simulink model "sampleModel2019_4_sub_sub_sub"  (R2023a)
settings: Solver=VariableStepAuto  StartTime=0.0  StopTime=10.0  RelTol=1e-3
libraries: hdlsllib x6, simulink x2
settings Model: Creator=user1  LastModifiedBy=user1
settings OptimizationCC: BlockReduction=off  ConditionallyExecuteInputs=off

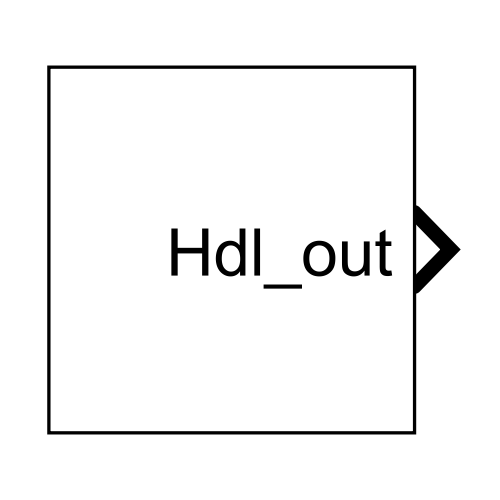
[thumbnail: Simulink's stored preview of the top-level diagram]
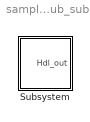
== system sampleModel2019_4_sub_sub_sub ==
  Subsystem : Subsystem

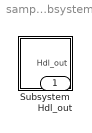
== system sampleModel2019_4_sub_sub_sub/Subsystem ==
  Subsystem : Subsystem
  Hdl_out : Outport  OutDataTypeStr=uint8

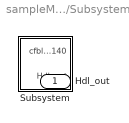
== system sampleModel2019_4_sub_sub_sub/Subsystem/Subsystem ==
  Subsystem : Subsystem
  Hdl_out : Outport  OutDataTypeStr=uint8

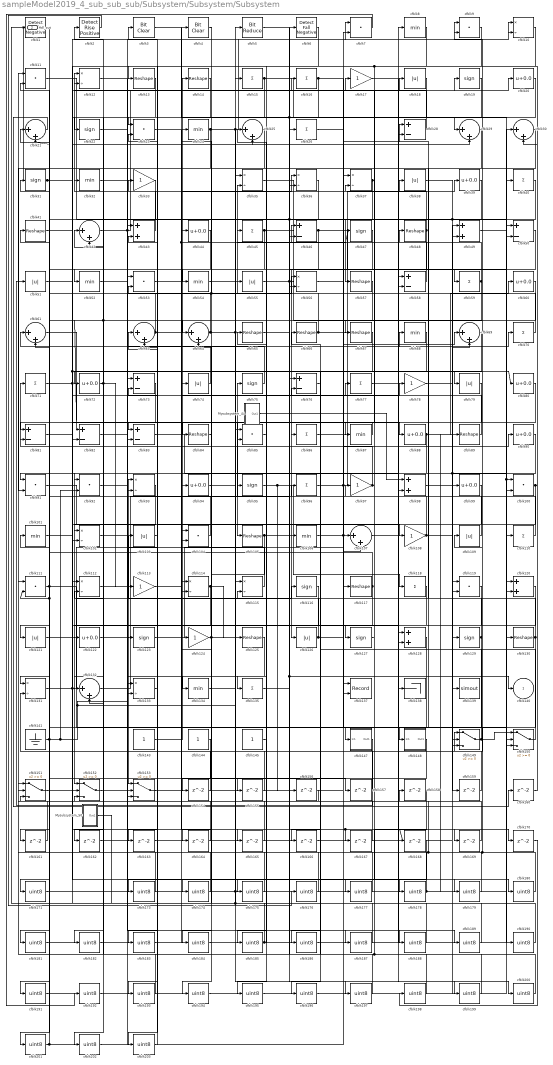
== system sampleModel2019_4_sub_sub_sub/Subsystem/Subsystem/Subsystem ==
  Mysubsystem_44 : Subsystem  TreatAsAtomicUnit=on  RTWFcnName=Mysubsystem_44
      settings: RTWFcnNameOpts=User specified  RTWFileNameOpts=Use function name
  Mysubsystem_50 : Subsystem  TreatAsAtomicUnit=on  RTWFcnName=Mysubsystem_50
      settings: RTWFcnNameOpts=User specified  RTWFileNameOpts=Use function name
  cfblk1 : hdlsllib/Logic and Bit Operations/Detect Fall Negative  vinit=0  OutDataTypeStr=uint8
  cfblk{10,12,35..37,56,93,102,112,114..115,131,133} (13 alike) : Product  Inputs=*/  OutDataTypeStr=uint8  RndMeth=Zero  SaturateOnIntegerOverflow=on
  cfblk{7,9,11,23,53,85,91..92,100,104,111,119} (12 alike) : DotProduct  OutDataTypeStr=uint8
  cfblk{8,24,32,52,54,68,87,101,106,134} (10 alike) : MinMax  OutDataTypeStr=uint8
  cfblk{18,38,51,55,74,79,103,109,121,126} (10 alike) : Abs  OutDataTypeStr=uint8  SaturateOnIntegerOverflow=off
  cfblk{13..14,41,48,57,65..67,84,89,105,117,125,130} (14 alike) : Reshape
  cfblk{21,25,29..30,42,61,63..64,69,107,132} (11 alike) : Sum  Inputs=|++  OutDataTypeStr=uint8
  cfblk{17,33,78,97,108,113,124} (7 alike) : Gain  OutDataTypeStr=uint8
  cfblk{15..16,26,40,45,59,70..71,77,86,96,110,118,135} (14 alike) : Sum  Inputs=+  OutDataTypeStr=uint8
  cfblk{19,22,31,47,75,95,116,123,127,129} (10 alike) : Signum
  cfblk{43,49,98,120,128} (5 alike) : Sum  OutDataTypeStr=uint8
  cfblk{20,39,44,60,72,80,88,90,94,99,122} (11 alike) : Bias  Bias=0.0  SaturateOnIntegerOverflow=off
  cfblk137 : Record  FileSettingsInternal="{\"entries\":[{\"content\":{\"excelSettings\":{\"content\":{},\"type\":\"Streamout.ExcelSettings\"}},\"type\":\"Streamout.FileSettingStorage\",\"uuid\":\"\"}],\"packageUris\":[\"http:\\/\\/schema.mathworks.com\\/mf0\\/streamout_blocks\\/R2020a\"],\"version\":\"1.0\"}"  Layout=[1 1]  SignalsInternal="{\"entries\":[{\"content\":{\"signals\":[{\"content\":{\"blockPath\":[],\"dimensions\":[1],\"domain\":\"\",\"lineColor\":\"#a2142f\",\"plots\":[1],\"port\":1,\"signalID\":59125,\"signalName\":\"cfblk55\"},\"type\":\"RecordBlkView.Signal\",\"uuid\":\"\"},{\"content\":{\"blockPath\":[],\"dimensions\":[1],\"domain\":\"\",\"lineColor\":\"#139fff\",\"plots\":[1],\"port\":2,\"signalID\":59128,\"signalName\":\"cfblk65\"},\"type\":\"RecordBlkView.Signal\",\"uuid\":\"\"}]},\"type\":\"RecordBlkView.InputSignals\",\"uuid\":\"\"}],\"packageUris\":[\"http:\\/\\/schema.mathworks.com\\/mf0\\/streamout_blocks\\/R2020a\"],\"version\":\"1.0\"}"  VisualizationBindings="{\"xyplotplugin\":{\"info\":[{\"series\":[{\"bindingParametersList\":[{\"parameter\":\"X-Axis\",\"signalID\":59125,\"signalName\":\"cfblk55\"},{\"parameter\":\"Y-Axis\",\"signalID\":59128,\"signalName\":\"cfblk65\"}],\"seriesID\":46600}],\"subplotID\":1}]}}"  CompatibilityTag=XY  st=-1
  cfblk138 : Terminator
  cfblk139 : ToWorkspace  VariableName=simout  SaveFormat=Timeseries  SampleTime=-1
  cfblk141 : Ground
  cfblk143 : Constant  OutDataTypeStr=uint8  SampleTime=-1
  cfblk144 : Constant  OutDataTypeStr=uint8  SampleTime=-1
  cfblk145 : Constant  OutDataTypeStr=uint8  SampleTime=-1
  cfblk147 : Subsystem
      settings: LibrarySourceBlock=|
      | hdlsllib/Ports &
      | Subsystems/Subsystem
  cfblk148 : Subsystem
      settings: LibrarySourceBlock=|
      | hdlsllib/Ports &
      | Subsystems/Subsystem
  cfblk{149..153} (5 alike) : Switch  OutDataTypeStr=uint8  SaturateOnIntegerOverflow=off  InputSameDT=off
  cfblk{154..170} (17 alike) : Delay  SampleTime=1
  cfblk{171,173..203} (32 alike) : DataTypeConversion  OutDataTypeStr=uint8  SaturateOnIntegerOverflow=off  RndMeth=Floor
  cfblk2 : hdlsllib/Logic and Bit Operations/Detect Rise Positive  vinit=0  OutDataTypeStr=uint8
  cfblk{28,46,50,58,73,76,81..83} (9 alike) : Sum  Inputs=+-  OutDataTypeStr=uint8
  cfblk3 : simulink/Logic and Bit Operations/Bit Clear  iBit=0
      settings: LibrarySourceBlock=|
      | hdlsllib/Logic and Bit
      | Operations/Bit Clear
  cfblk4 : simulink/Logic and Bit Operations/Bit Clear  iBit=0
      settings: LibrarySourceBlock=|
      | hdlsllib/Logic and Bit
      | Operations/Bit Clear
  cfblk5 : hdlsllib/Logic and Bit Operations/Bit Reduce  mode=AND
  cfblk6 : hdlsllib/Logic and Bit Operations/Detect Fall Negative  vinit=0  OutDataTypeStr=uint8
  cfblk140 : Outport  OutDataTypeStr=uint8  VectorParamsAs1DForOutWhenUnconnected=off
  Hdl_out : Outport  Port=2  OutDataTypeStr=uint8
  wires:
  cfblk95/1 -> cfblk156/1, cfblk118/1
  cfblk75/1 -> cfblk61/1
  cfblk40/1 -> cfblk149/2, cfblk152/1
  cfblk109/1 -> cfblk31/1
  cfblk100/1 -> cfblk134/1, cfblk13/1
  cfblk115/1 -> cfblk14/1
  cfblk101/1 -> cfblk178/1
  cfblk114/1 -> cfblk162/1, cfblk125/1
  cfblk112/1 -> cfblk187/1
  cfblk96/1 -> cfblk28/1, cfblk39/1
  cfblk66/1 -> cfblk38/1, cfblk24/1, cfblk21/1
  cfblk104/1 -> cfblk44/1
  cfblk42/1 -> cfblk108/1, cfblk20/1
  cfblk11/1 -> cfblk57/1
  cfblk116/1 -> cfblk135/1
  cfblk143/1 -> cfblk104/1
  cfblk126/1 -> cfblk150/2, cfblk93/1
  cfblk58/1 -> cfblk35/2
  cfblk105/1 -> cfblk194/1, cfblk179/1
  cfblk43/1 -> cfblk12/1
  cfblk25/1 -> cfblk64/1
  cfblk93/1 -> cfblk102/1
  cfblk47/1 -> cfblk121/1
  cfblk131/1 -> cfblk170/1, cfblk94/1
  cfblk88/1 -> cfblk195/1, cfblk60/1
  cfblk46/1 -> cfblk114/2, cfblk120/1
  cfblk50/1 -> cfblk126/1
  cfblk39/1 -> cfblk46/2, cfblk52/1
  cfblk110/1 -> cfblk96/1
  cfblk8/1 -> cfblk185/1
  cfblk64/1 -> cfblk2/1, cfblk46/1, cfblk79/1
  cfblk63/1 -> cfblk42/2, cfblk36/1
  cfblk9/1 -> cfblk23/1
  cfblk83/1 -> cfblk138/1
  cfblk90/1 -> cfblk131/1
  cfblk107/1 -> cfblk180/1
  cfblk15/1 -> cfblk110/1, cfblk83/1
  cfblk106/1 -> cfblk140/1, cfblk69/1
  cfblk102/1 -> cfblk153/1
  cfblk121/1 -> cfblk26/1
  cfblk57/1 -> cfblk182/1, cfblk82/1
  cfblk149/1 -> cfblk150/1, cfblk66/1
  cfblk134/1 -> cfblk116/1
  cfblk127/1 -> cfblk97/1
  cfblk147/1(Out1) -> cfblk51/1
  cfblk24/1 -> cfblk91/2, cfblk128/2, cfblk7/1
  cfblk141/1 -> cfblk21/2, cfblk92/2, cfblk15/1, cfblk53/1
  cfblk10/1 -> cfblk67/1, cfblk102/2
  cfblk26/1 -> cfblk59/1
  cfblk35/1 -> cfblk130/1
  cfblk153/1 -> cfblk7/2
  cfblk92/1 -> cfblk56/1
  cfblk120/1 -> cfblk153/2
  cfblk130/1 -> cfblk63/2, cfblk149/1
  cfblk17/1 -> cfblk128/1
  cfblk60/1 -> cfblk120/2
  cfblk132/1 -> cfblk6/1
  cfblk59/1 -> cfblk28/2, cfblk91/1
  cfblk12/1 -> cfblk86/1
  cfblk86/1 -> cfblk70/1
  cfblk61/1 -> cfblk106/1
  cfblk145/1 -> cfblk25/1
  cfblk54/1 -> cfblk5/1
  cfblk123/1 -> cfblk90/1
  cfblk32/1 -> cfblk9/1
  cfblk14/1 -> cfblk82/2
  cfblk70/1 -> cfblk45/1
  cfblk82/1 -> cfblk168/1, cfblk167/1
  cfblk78/1 -> cfblk100/2, cfblk129/1
  cfblk73/1 -> cfblk201/1
  cfblk31/1 -> Hdl_out/1, cfblk104/2
  cfblk79/1 -> cfblk83/2
  cfblk1/1 -> cfblk171/1
  cfblk20/1 -> cfblk22/1
  cfblk28/1 -> cfblk12/2
  cfblk30/1 -> cfblk72/1
  cfblk29/1 -> cfblk148/1(In1)
  cfblk91/1 -> cfblk114/1
  cfblk37/1 -> cfblk132/2, cfblk87/1
  cfblk111/1 -> cfblk11/2, cfblk147/1(In1)
  cfblk41/1 -> cfblk127/1, cfblk80/1
  cfblk18/1 -> cfblk98/2
  cfblk97/1 -> cfblk17/1, cfblk71/1
  cfblk80/1 -> cfblk105/1
  cfblk98/1 -> cfblk99/1
  cfblk3/1 -> cfblk29/1
  cfblk152/1 -> cfblk68/1
  cfblk44/1 -> cfblk93/2
  cfblk22/1 -> cfblk19/1
  cfblk129/1 -> cfblk186/1, cfblk48/1
  cfblk89/1 -> cfblk74/1
  cfblk108/1 -> cfblk69/2, cfblk53/2
  cfblk52/1 -> cfblk29/2
  cfblk122/1 -> cfblk75/1
  cfblk68/1 -> cfblk84/1
  cfblk55/1 -> cfblk197/1, cfblk137/1
  cfblk48/1 -> cfblk54/1, cfblk3/1
  cfblk76/1 -> cfblk196/1
  cfblk56/1 -> cfblk10/1
  cfblk74/1 -> cfblk23/2
  cfblk72/1 -> cfblk202/1, cfblk113/1
  cfblk144/1 -> cfblk152/2
  cfblk65/1 -> cfblk189/1, cfblk137/2
  cfblk13/1 -> cfblk122/1
  cfblk71/1 -> cfblk88/1, cfblk18/1
  cfblk16/1 -> cfblk150/3, cfblk36/2, cfblk92/1
  cfblk81/1 -> cfblk25/2
  cfblk45/1 -> cfblk139/1, cfblk123/1
  cfblk133/1 -> cfblk43/2
  cfblk6/1 -> cfblk56/2
  cfblk151/1 -> cfblk78/1
  cfblk113/1 -> cfblk16/1, cfblk47/1
  cfblk125/1 -> cfblk153/3
  cfblk69/1 -> cfblk132/1
  cfblk124/1 -> cfblk174/1, cfblk169/1
  cfblk77/1 -> cfblk199/1
  cfblk87/1 -> cfblk81/1
  cfblk150/1 -> cfblk109/1
  cfblk5/1 -> cfblk50/2, cfblk58/2
  cfblk51/1 -> cfblk10/2
  cfblk117/1 -> cfblk61/2, cfblk133/2
  cfblk84/1 -> cfblk154/1
  cfblk154/1 -> cfblk131/2
  cfblk118/1 -> cfblk155/1
  cfblk155/1 -> cfblk133/1
  cfblk156/1 -> cfblk151/3
  cfblk23/1 -> cfblk157/1
  cfblk157/1 -> cfblk81/2
  cfblk38/1 -> cfblk159/1
  cfblk159/1 -> cfblk35/1
  cfblk21/1 -> cfblk160/1
  cfblk160/1 -> cfblk30/2
  cfblk128/1 -> cfblk161/1
  cfblk161/1 -> cfblk151/2
  cfblk162/1 -> cfblk149/3
  cfblk36/1 -> cfblk163/1
  cfblk163/1 -> cfblk37/1
  cfblk19/1 -> cfblk164/1
  cfblk164/1 -> cfblk42/1
  cfblk53/1 -> cfblk165/1
  cfblk165/1 -> cfblk63/1
  cfblk67/1 -> cfblk166/1
  cfblk166/1 -> cfblk58/1
  cfblk167/1 -> cfblk43/1
  cfblk169/1 -> cfblk64/2
  cfblk171/1 -> cfblk55/1, cfblk50/1
  cfblk103/1 -> cfblk173/1
  cfblk173/1 -> cfblk32/1
  cfblk174/1 -> cfblk103/1
  cfblk85/1 -> cfblk175/1
  cfblk175/1 -> cfblk151/1
  cfblk2/1 -> cfblk176/1
  cfblk176/1 -> cfblk85/1
  cfblk158/1 -> cfblk177/1
  cfblk177/1 -> cfblk85/2
  cfblk178/1 -> cfblk89/1, cfblk115/2
  cfblk179/1 -> cfblk101/1
  cfblk180/1 -> cfblk9/2, cfblk33/1, cfblk158/1
  cfblk148/1(Out1) -> cfblk181/1
  cfblk181/1 -> cfblk107/1
  cfblk182/1 -> cfblk107/2
  cfblk99/1 -> cfblk183/1
  cfblk183/1 -> cfblk4/1
  cfblk4/1 -> cfblk184/1
  cfblk184/1 -> cfblk40/1
  cfblk185/1 -> cfblk65/1, cfblk11/1
  cfblk186/1 -> cfblk8/1
  cfblk187/1 -> cfblk115/1, cfblk124/1
  cfblk135/1 -> cfblk188/1
  cfblk188/1 -> cfblk112/1
  cfblk189/1 -> cfblk112/2
  cfblk49/1 -> cfblk190/1
  cfblk190/1 -> cfblk95/1
  cfblk33/1 -> cfblk191/1
  cfblk191/1 -> cfblk49/1
  cfblk7/1 -> cfblk192/1
  cfblk192/1 -> cfblk49/2
  cfblk119/1 -> cfblk193/1
  cfblk193/1 -> cfblk111/1
  cfblk194/1 -> cfblk119/1
  cfblk195/1 -> cfblk119/2
  cfblk196/1 -> cfblk30/1, cfblk100/1
  cfblk197/1 -> cfblk76/1
  cfblk170/1 -> cfblk198/1
  cfblk198/1 -> cfblk76/2
  cfblk199/1 -> cfblk152/3, cfblk37/2
  cfblk94/1 -> cfblk200/1
  cfblk200/1 -> cfblk77/1
  cfblk201/1 -> cfblk117/1, cfblk111/2, cfblk41/1
  cfblk202/1 -> cfblk73/1
  cfblk168/1 -> cfblk203/1
  cfblk203/1 -> cfblk73/2
  Mysubsystem_44/1(Out1) -> cfblk98/1
  Mysubsystem_50/1(Out1) -> cfblk1/1

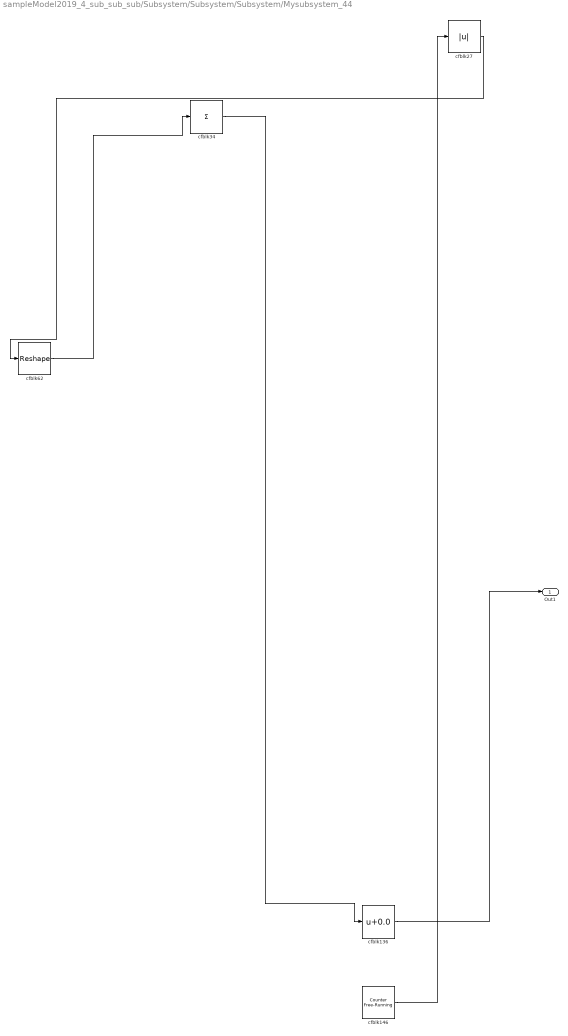
== system sampleModel2019_4_sub_sub_sub/Subsystem/Subsystem/Subsystem/Mysubsystem_44 ==
  cfblk136 : Bias  Bias=0.0  SaturateOnIntegerOverflow=off
  cfblk146 : hdlsllib/Sources/Counter Free-Running  NumBits=16  tsamp=-1
  cfblk27 : Abs  SaturateOnIntegerOverflow=off
  cfblk34 : Sum  Inputs=+
  cfblk62 : Reshape
  Out1 : Outport
  wires:
  cfblk62/1 -> cfblk34/1
  cfblk146/1 -> cfblk27/1
  cfblk34/1 -> cfblk136/1
  cfblk27/1 -> cfblk62/1
  cfblk136/1 -> Out1/1

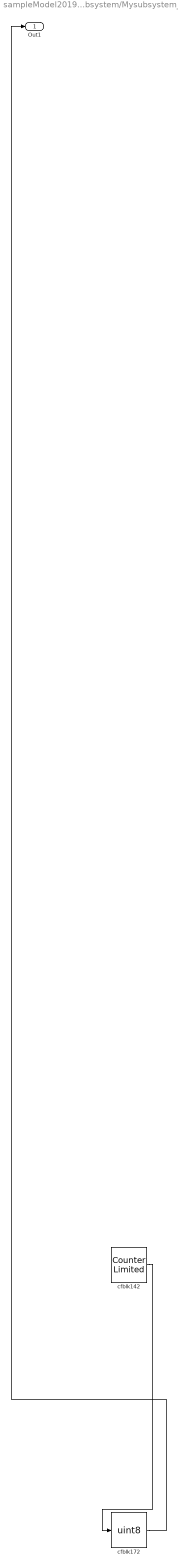
== system sampleModel2019_4_sub_sub_sub/Subsystem/Subsystem/Subsystem/Mysubsystem_50 ==
  cfblk142 : hdlsllib/Sources/Counter Limited  uplimit=7  tsamp=-1
  cfblk172 : DataTypeConversion  OutDataTypeStr=uint8  SaturateOnIntegerOverflow=off  RndMeth=Floor
  Out1 : Outport
  wires:
  cfblk172/1 -> Out1/1
  cfblk142/1 -> cfblk172/1

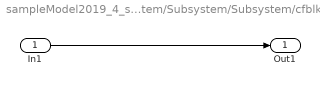
== system sampleModel2019_4_sub_sub_sub/Subsystem/Subsystem/Subsystem/cfblk147 ==
  In1 : Inport
  Out1 : Outport
  wires:
  In1/1 -> Out1/1

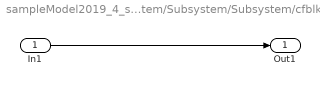
== system sampleModel2019_4_sub_sub_sub/Subsystem/Subsystem/Subsystem/cfblk148 ==
  In1 : Inport
  Out1 : Outport
  wires:
  In1/1 -> Out1/1
